simulink model "IMC_datta_20140127"  (Simulink 7.9)
settings: Solver=ode45  StartTime=0.0  StopTime=20  FixedStep=Ts  RelTol=1e-3
InitFcn:
  | IMC_datta_ini
values from neighbouring files (symbols this model uses):
  Ts = 0.5    [IMC_calculo_limites_thetas.m]    (also in IMC_datta_ini.m; IMC_ini.m = 8.33333333333e-05; JORGE_controlador_LCL_malha_interna.m = 8.33333333333e-05; LCL_PAPM.m = 8.33333333333e-05)
undefined symbols (not defined in the file or in its folder): PD, PN
settings Model: Creator=Marcelo  LastModifiedBy=marcelodurgante
settings OptimizationCC: ExpressionDepthLimit=128
settings CodeAppCC: CustomSymbolStrType=$N$R$M_T
settings GRTTargetCC: CombineOutputUpdateFcns=off  GRTInterface=on

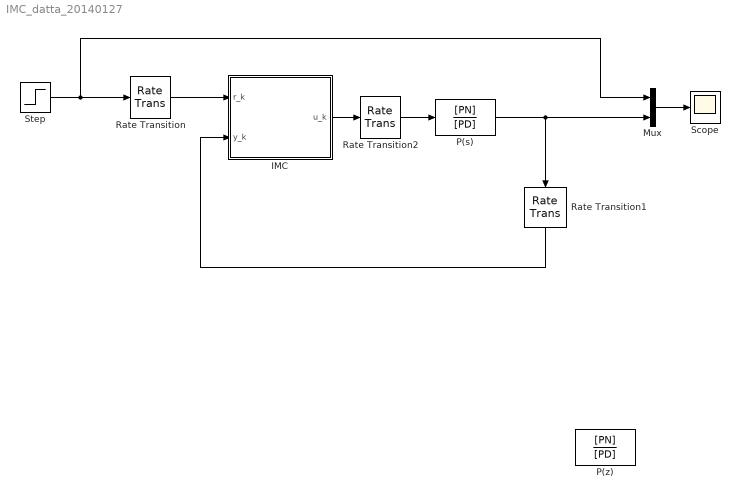
== system IMC_datta_20140127 ==
  IMC : MATLAB Function  TreatAsAtomicUnit=on
  Mux : Mux  Inputs=2
  P(s) : TransferFcn  Numerator=[PN]  Denominator=[PD]
  P(z) : DiscreteTransferFcn  Numerator=[PN]  Denominator=[PD]  SampleTime=Ts
  Rate Transition : RateTransition  OutPortSampleTime=Ts
  Rate Transition1 : RateTransition  OutPortSampleTime=Ts
  Rate Transition2 : RateTransition  OutPortSampleTime=Ts
  Scope : Scope
      settings: YMin=-1.5  YMax=2
  Step : Step  Time=2  SampleTime=0
  wires:
  P(s)/1 -> Rate Transition1/1, Mux/2
  Mux/1 -> Scope/1
  Step/1 -> Rate Transition/1, Mux/1
  Rate Transition2/1 -> P(s)/1
  IMC/1(u_k) -> Rate Transition2/1
  Rate Transition/1 -> IMC/1(r_k)
  Rate Transition1/1 -> IMC/2(y_k)

== matlab function IMC ==
  data: r_k input double; y_k input double; u_k output double
function u_k = imc(r_k, y_k)
%#CODEGEN

%ganho adaptativo entre 0 e 0.5
gamma=0.4;

%constante escolhida entre 0 e 1
delta0=0.36;

%lambdas escolhidos de forma que Lambda seja estável
lambda0=-0.1;
lambda1=-0.02;

%definição do conjunto no qual serão projetados os parâmetros
theta1_min= 0.4;
theta1_max= 1.2;
theta2_min= -1;
theta2_max= -0.1;
theta3_min= -0.18;
theta3_max= -0.05;
theta4_min= 0.2;
theta4_max= 1;

%l é o grau do numerador e n é o grau do denominador da parte modelada da
%planta

%% Declarações

persistent theta_k;
if isempty(theta_k)
    theta_k=[0.8744; -0.2431; -0.1612; 0.2856];
end

persistent phi11_k1;
if isempty(phi11_k1)
    phi11_k1=0;
end

persistent phi11_k2;
if isempty(phi11_k2)
    phi11_k2=0;
end

persistent phi12_k1;
if isempty(phi12_k1)
    phi12_k1=0;
end

persistent phi12_k2;
if isempty(phi12_k2)
    phi12_k2=0;
end

persistent phi21_k1;
if isempty(phi21_k1)
    phi21_k1=0;
end

persistent phi21_k2;
if isempty(phi21_k2)
    phi21_k2=0;
end

persistent phi22_k1;
if isempty(phi22_k1)
    phi22_k1=0;
end

persistent phi22_k2;
if isempty(phi22_k2)
    phi22_k2=0;
end

persistent u_k1;
if isempty(u_k1)
    u_k1=0;
end

persistent u_k2;
if isempty(u_k2)
    u_k2=0;
end

persistent y_k1;
if isempty(y_k1)
    y_k1=0;
end

persistent y_k2;
if isempty(y_k2)
    y_k2=0;
end

persistent rer_k1;
if isempty(rer_k1)
    rer_k1=0;
end

persistent rer_k2;
if isempty(rer_k2)
    rer_k2=0;
end

persistent m2;
if isempty(m2)
    m2=1;
end

%% Cálculos

phi11_k = y_k1 - lambda1*phi11_k1 - lambda0*phi11_k2;
phi12_k = y_k2 - lambda1*phi12_k1 - lambda0*phi12_k2;
phi21_k = u_k1 - lambda1*phi21_k1 - lambda0*phi21_k2;
phi22_k = u_k2 - lambda1*phi22_k1 - lambda0*phi22_k2;

phi1_k=[phi11_k phi12_k];
phi2_k=[phi21_k phi22_k];

phi_k = [phi1_k'; phi2_k'];

m2_k= m2 + phi_k'*phi_k;

y_hat_k= theta_k'*phi_k;

eta_k= (y_k - y_hat_k)/m2_k;

% Ação de Controle
rer_k = r_k - (y_k - y_hat_k);
phi = - theta_k(3)/theta_k(4);
ganho = (1-phi)/(theta_k(3)+theta_k(4));

u_k = ganho*(rer_k + (lambda1-theta_k(1))*rer_k1 + (lambda0-theta_k(2))*rer_k2) + phi*u_k1;



%% Atualização

m2 = delta0*(m2 - 1) + u_k^2 + y_k^2 + 1;

%atualização de theta_k via algoritmo de projeção de parâmetros
g1_k= -gamma*eta_k*phi11_k;
g2_k= -gamma*eta_k*phi12_k;
g3_k= -gamma*eta_k*phi21_k;
g4_k= -gamma*eta_k*phi22_k;

f1_k=0;
if (theta_k(1)+g1_k)>theta1_max
    f1_k=theta1_max-theta_k(1)-g1_k;
end
if (theta_k(1)+g1_k)<theta1_min
    f1_k=theta1_min-theta_k(1)-g1_k;
end

f2_k=0;
if (theta_k(2)+g2_k)>theta2_max
    f2_k=theta2_max-theta_k(2)-g2_k;
end
if (theta_k(2)+g2_k)<theta2_min
    f2_k=theta2_min-theta_k(2)-g2_k;
end

f3_k=0;
if (theta_k(3)+g3_k)>theta3_max
    f3_k=theta3_max-theta_k(3)-g3_k;
end
if (theta_k(3)+g3_k)<theta3_min
    f3_k=theta3_min-theta_k(3)-g3_k;
end

f4_k=0;
if (theta_k(4)+g4_k)>theta4_max
    f4_k=theta4_max-theta_k(4)-g4_k;
end
if (theta_k(4)+g4_k)<theta4_min
    f4_k=theta4_min-theta_k(4)-g4_k;
end

f_k = [f1_k; f2_k; f3_k; f4_k];

theta_k = theta_k + gamma*eta_k*phi_k + f_k;


%atualização de estados anteriores
phi11_k2 = phi11_k1;
phi11_k1 = phi11_k;
phi12_k2 = phi12_k1;
phi12_k1 = phi12_k;
phi21_k2 = phi21_k1;
phi21_k1 = phi21_k;
phi22_k2 = phi22_k1;
phi22_k1 = phi22_k;

u_k2 = u_k1;
u_k1 = u_k;

y_k2 = y_k1;
y_k1 = y_k;

rer_k2 = rer_k1;
rer_k1 = rer_k;


end
